simulink model "dsb_sys"  (R2019b)
settings: Solver=VariableStepAuto  StartTime=0.0  StopTime=3  RelTol=1e-3
libraries: commanapbnd3 x2
settings Model: Creator=yango  LastModifiedBy=yango

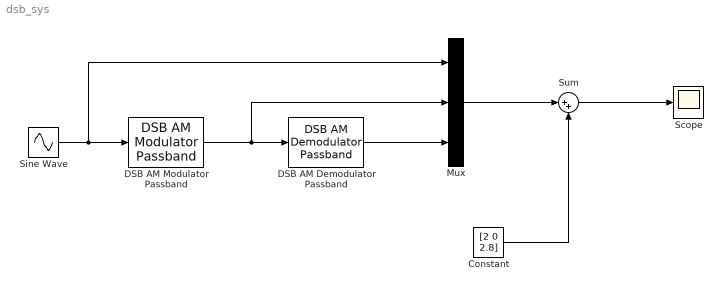
== system dsb_sys ==
  Constant : Constant  Value=[2 0 2.8]
  DSB AM Demodulator Passband : commanapbnd3/DSB AM Demodulator Passband  Fc=180  Ph=pi/3  method=Butterworth  n=4  cf=16  Rp=0.1  Rs=50  Offset=1
      settings: SourceProductName=Communications Toolbox  SourceProductBaseCode=CM
  DSB AM Modulator Passband : commanapbnd3/DSB AM Modulator Passband  Fc=180  Ph=pi/3  Offset=1
      settings: SourceProductName=Communications Toolbox  SourceProductBaseCode=CM
  Mux : Mux  Inputs=3
  Scope : Scope
  Sine Wave : Sin  Amplitude=0.7  Frequency=8  SampleTime=0.01
  Sum : Sum  Inputs=|++
  wires:
  DSB AM Modulator Passband/1 -> Mux/2, DSB AM Demodulator Passband/1
  Sine Wave/1 -> Mux/1, DSB AM Modulator Passband/1
  DSB AM Demodulator Passband/1 -> Mux/3
  Constant/1 -> Sum/2
  Mux/1 -> Sum/1
  Sum/1 -> Scope/1
